simulink model "naibaoDSTBC_42"  (R2018a)
settings: Solver=VariableStepAuto  StartTime=0.0  StopTime=1  RelTol=1e-3
model workspace (MAT data in the model file):
  FrameLength = 100
  SampleTime = 0.001
  maxNumBits = 100000000
  maxNumErrs = 1000
undefined symbols (not defined in the file): doppler
libraries: commchan3 x9, commrandsrc3 x1, commsink2 x1
settings Model: Creator=myste  LastModifiedBy=myste

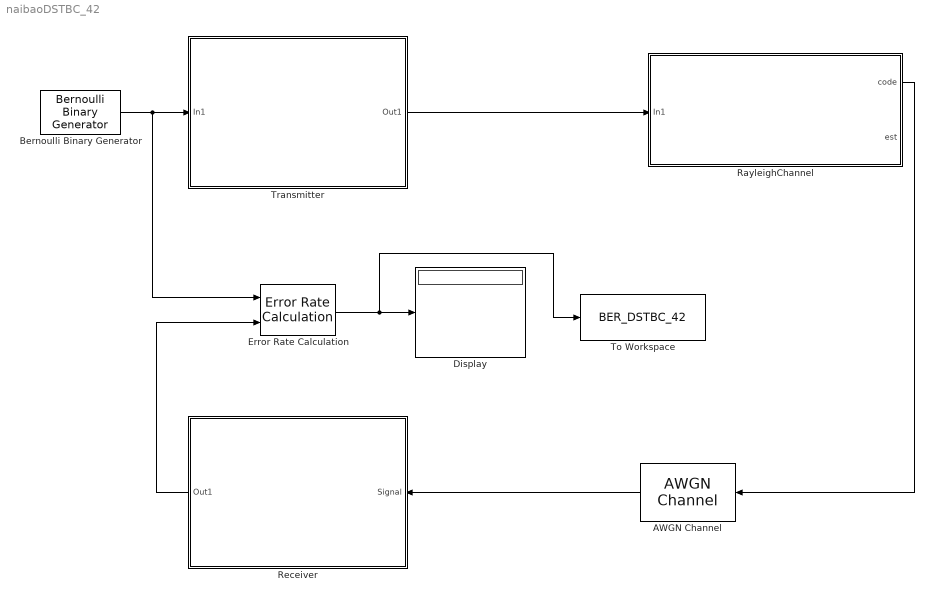
== system naibaoDSTBC_42 ==
  AWGN Channel : commchan3/AWGN Channel  InputProcessing=Columns as channels (frame based)  seed=3472  noiseMode="Signal to noise ratio  (Eb/No)"  EbNodB=EbNo  EsNodB=10  SNRdB=10  bitsPerSym=1  Ps=1  Tsym=SampleTime*1/2  variance=1
  Bernoulli Binary Generator : commrandsrc3/Bernoulli Binary Generator  ProbabilityOfZero=0.5  SeedSource=Auto  Seed=1983  SampleTime=SampleTime  SamplesPerFrame=FrameLength  OutputDataType=boolean  SimulateUsing=Interpreted execution
  Display : Display
  Error Rate Calculation : commsink2/Error Rate Calculation  N=0  st_delay=0  cp_mode=Entire frame  subframe=[]  PMode=Port  WsName=ErrorVec  RsMode2=off  stop=on  numErr=maxNumErrs  maxBits=maxNumBits
  RayleighChannel : Subsystem
  Receiver : Subsystem
  To Workspace : ToWorkspace  VariableName=BER_DSTBC_42  SampleTime=-1
      settings: MaxDataPoints=1  Save2DSignal=2-D array (concatenate along first dimension)
  Transmitter : Subsystem
  wires:
  Bernoulli Binary Generator/1 -> Error Rate Calculation/1, Transmitter/1(In1)
  Transmitter/1(Out1) -> RayleighChannel/1(In1)
  Receiver/1(Out1) -> Error Rate Calculation/2
  Error Rate Calculation/1 -> To Workspace/1, Display/1
  RayleighChannel/1(code) -> AWGN Channel/1
  AWGN Channel/1 -> Receiver/1(Signal)

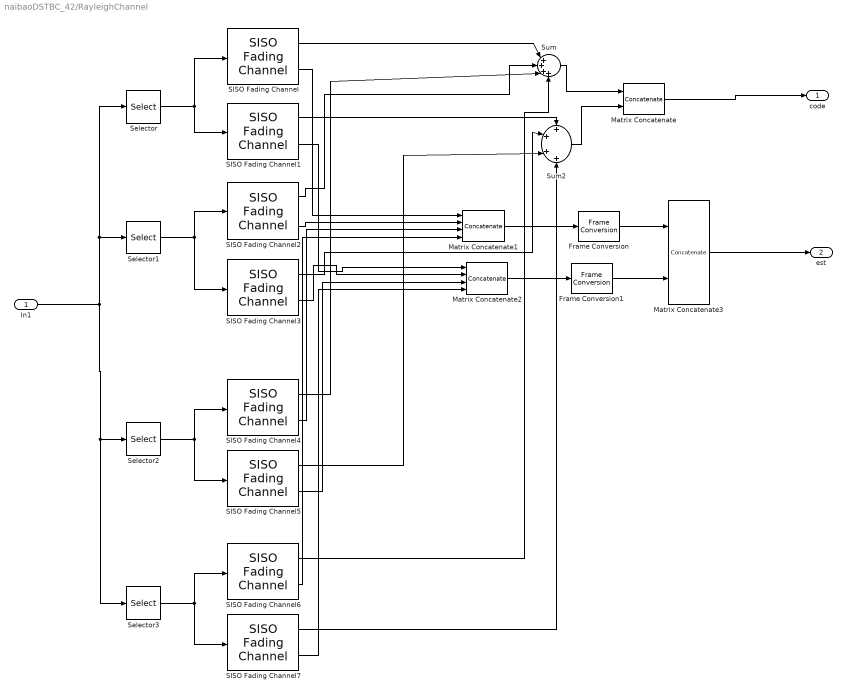
== system naibaoDSTBC_42/RayleighChannel ==
  In1 : Inport
  Frame Conversion : FrameConversion  OutFrame=Sample-based
  Frame Conversion1 : FrameConversion  OutFrame=Sample-based
  Matrix Concatenate : Concatenate  Mode=Multidimensional array  ConcatenateDimension=2
  Matrix Concatenate1 : Concatenate  NumInputs=4  Mode=Multidimensional array  ConcatenateDimension=2
  Matrix Concatenate2 : Concatenate  NumInputs=4  Mode=Multidimensional array  ConcatenateDimension=2
  Matrix Concatenate3 : Concatenate  Mode=Multidimensional array  ConcatenateDimension=3
  SISO Fading Channel : commchan3/SISO Fading Channel  InheritSampleRate=on  SampleRate=1  PathDelays=0  AveragePathGains=0  NormalizePathGains=on  FadingDistribution=Rayleigh  KFactor=3  DirectPathDopplerShift=0  DirectPathInitialPhase=0  MaximumDopplerShift=3  DopplerSpectrum=doppler('Jakes')  ChannelInterpolationMethod=Polyphase  RandomStream=mt19937ar with seed  RandomNumGenerator=mt19937ar  Seed=123  PathGainsOutputPort=on  ChannelFilterDelayOutputPort=off  SimulateUsing=Interpreted execution  Visualization=Off  PathsForDopplerDisplay=1  SamplesToDisplay=25%
      settings: SourceProductName=Communications System Toolbox
  SISO Fading Channel1 : commchan3/SISO Fading Channel  InheritSampleRate=on  SampleRate=1  PathDelays=0  AveragePathGains=0  NormalizePathGains=on  FadingDistribution=Rayleigh  KFactor=3  DirectPathDopplerShift=0  DirectPathInitialPhase=0  MaximumDopplerShift=3  DopplerSpectrum=doppler('Jakes')  ChannelInterpolationMethod=Polyphase  RandomStream=mt19937ar with seed  RandomNumGenerator=mt19937ar  Seed=73  PathGainsOutputPort=on  ChannelFilterDelayOutputPort=off  SimulateUsing=Interpreted execution  Visualization=Off  PathsForDopplerDisplay=1  SamplesToDisplay=25%
      settings: SourceProductName=Communications System Toolbox
  SISO Fading Channel2 : commchan3/SISO Fading Channel  InheritSampleRate=on  SampleRate=1  PathDelays=0  AveragePathGains=0  NormalizePathGains=on  FadingDistribution=Rayleigh  KFactor=3  DirectPathDopplerShift=0  DirectPathInitialPhase=0  MaximumDopplerShift=3  DopplerSpectrum=doppler('Jakes')  ChannelInterpolationMethod=Polyphase  RandomStream=mt19937ar with seed  RandomNumGenerator=mt19937ar  Seed=88  PathGainsOutputPort=on  ChannelFilterDelayOutputPort=off  SimulateUsing=Interpreted execution  Visualization=Off  PathsForDopplerDisplay=1  SamplesToDisplay=25%
      settings: SourceProductName=Communications System Toolbox
  SISO Fading Channel3 : commchan3/SISO Fading Channel  InheritSampleRate=on  SampleRate=1  PathDelays=0  AveragePathGains=0  NormalizePathGains=on  FadingDistribution=Rayleigh  KFactor=3  DirectPathDopplerShift=0  DirectPathInitialPhase=0  MaximumDopplerShift=3  DopplerSpectrum=doppler('Jakes')  ChannelInterpolationMethod=Polyphase  RandomStream=mt19937ar with seed  RandomNumGenerator=mt19937ar  Seed=95  PathGainsOutputPort=on  ChannelFilterDelayOutputPort=off  SimulateUsing=Interpreted execution  Visualization=Off  PathsForDopplerDisplay=1  SamplesToDisplay=25%
      settings: SourceProductName=Communications System Toolbox
  SISO Fading Channel4 : commchan3/SISO Fading Channel  InheritSampleRate=on  SampleRate=1  PathDelays=0  AveragePathGains=0  NormalizePathGains=on  FadingDistribution=Rayleigh  KFactor=3  DirectPathDopplerShift=0  DirectPathInitialPhase=0  MaximumDopplerShift=3  DopplerSpectrum=doppler('Jakes')  ChannelInterpolationMethod=Polyphase  RandomStream=mt19937ar with seed  RandomNumGenerator=mt19937ar  Seed=102  PathGainsOutputPort=on  ChannelFilterDelayOutputPort=off  SimulateUsing=Interpreted execution  Visualization=Off  PathsForDopplerDisplay=1  SamplesToDisplay=25%
      settings: SourceProductName=Communications System Toolbox
  SISO Fading Channel5 : commchan3/SISO Fading Channel  InheritSampleRate=on  SampleRate=1  PathDelays=0  AveragePathGains=0  NormalizePathGains=on  FadingDistribution=Rayleigh  KFactor=3  DirectPathDopplerShift=0  DirectPathInitialPhase=0  MaximumDopplerShift=3  DopplerSpectrum=doppler('Jakes')  ChannelInterpolationMethod=Polyphase  RandomStream=mt19937ar with seed  RandomNumGenerator=mt19937ar  Seed=143  PathGainsOutputPort=on  ChannelFilterDelayOutputPort=off  SimulateUsing=Interpreted execution  Visualization=Off  PathsForDopplerDisplay=1  SamplesToDisplay=25%
      settings: SourceProductName=Communications System Toolbox
  SISO Fading Channel6 : commchan3/SISO Fading Channel  InheritSampleRate=on  SampleRate=1  PathDelays=0  AveragePathGains=0  NormalizePathGains=on  FadingDistribution=Rayleigh  KFactor=3  DirectPathDopplerShift=0  DirectPathInitialPhase=0  MaximumDopplerShift=3  DopplerSpectrum=doppler('Jakes')  ChannelInterpolationMethod=Polyphase  RandomStream=mt19937ar with seed  RandomNumGenerator=mt19937ar  Seed=127  PathGainsOutputPort=on  ChannelFilterDelayOutputPort=off  SimulateUsing=Interpreted execution  Visualization=Off  PathsForDopplerDisplay=1  SamplesToDisplay=25%
      settings: SourceProductName=Communications System Toolbox
  SISO Fading Channel7 : commchan3/SISO Fading Channel  InheritSampleRate=on  SampleRate=1  PathDelays=0  AveragePathGains=0  NormalizePathGains=on  FadingDistribution=Rayleigh  KFactor=3  DirectPathDopplerShift=0  DirectPathInitialPhase=0  MaximumDopplerShift=3  DopplerSpectrum=doppler('Jakes')  ChannelInterpolationMethod=Polyphase  RandomStream=mt19937ar with seed  RandomNumGenerator=mt19937ar  Seed=164  PathGainsOutputPort=on  ChannelFilterDelayOutputPort=off  SimulateUsing=Interpreted execution  Visualization=Off  PathsForDopplerDisplay=1  SamplesToDisplay=25%
      settings: SourceProductName=Communications System Toolbox
  Selector : Selector  NumberOfDimensions=2  InputPortWidth=3  IndexOptions=Select all,Index vector (dialog)  Indices=[1 3],1  OutputSizes=1,1
  Selector1 : Selector  NumberOfDimensions=2  InputPortWidth=3  IndexOptions=Select all,Index vector (dialog)  Indices=[1 3],2  OutputSizes=1,1
  Selector2 : Selector  NumberOfDimensions=2  InputPortWidth=3  IndexOptions=Select all,Index vector (dialog)  Indices=[1 3],3  OutputSizes=1,1
  Selector3 : Selector  NumberOfDimensions=2  InputPortWidth=3  IndexOptions=Select all,Index vector (dialog)  Indices=[1 3],4  OutputSizes=1,1
  Sum : Sum  Inputs=|++++
  Sum2 : Sum  Inputs=++++
  code : Outport
  est : Outport  Port=2
  wires:
  In1/1 -> Selector3/1, Selector2/1, Selector/1, Selector1/1
  Selector/1 -> SISO Fading Channel/1, SISO Fading Channel1/1
  Selector1/1 -> SISO Fading Channel3/1, SISO Fading Channel2/1
  SISO Fading Channel/1 -> Sum/1
  SISO Fading Channel2/1 -> Sum/2
  SISO Fading Channel1/1 -> Sum2/1
  Sum/1 -> Matrix Concatenate/1
  Sum2/1 -> Matrix Concatenate/2
  SISO Fading Channel/2 -> Matrix Concatenate1/1
  SISO Fading Channel3/1 -> Sum2/2
  SISO Fading Channel2/2 -> Matrix Concatenate1/2
  SISO Fading Channel1/2 -> Matrix Concatenate2/1
  SISO Fading Channel3/2 -> Matrix Concatenate2/2
  Matrix Concatenate/1 -> code/1
  Matrix Concatenate1/1 -> Frame Conversion/1
  Matrix Concatenate2/1 -> Frame Conversion1/1
  Frame Conversion1/1 -> Matrix Concatenate3/2
  Frame Conversion/1 -> Matrix Concatenate3/1
  Matrix Concatenate3/1 -> est/1
  Selector2/1 -> SISO Fading Channel5/1, SISO Fading Channel4/1
  Selector3/1 -> SISO Fading Channel6/1, SISO Fading Channel7/1
  SISO Fading Channel4/1 -> Sum/3
  SISO Fading Channel6/1 -> Sum/4
  SISO Fading Channel5/1 -> Sum2/3
  SISO Fading Channel7/1 -> Sum2/4
  SISO Fading Channel4/2 -> Matrix Concatenate1/3
  SISO Fading Channel6/2 -> Matrix Concatenate1/4
  SISO Fading Channel5/2 -> Matrix Concatenate2/3
  SISO Fading Channel7/2 -> Matrix Concatenate2/4

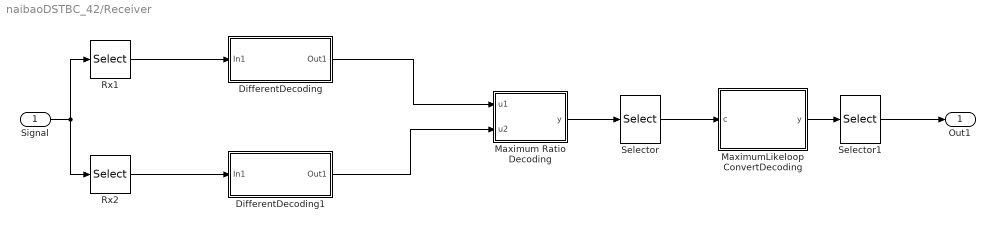
== system naibaoDSTBC_42/Receiver ==
  Signal : Inport
  DifferentDecoding : Subsystem
  DifferentDecoding1 : Subsystem
  Maximum Ratio Decoding : MATLAB Function  TreatAsAtomicUnit=on
  MaximumLikeloop ConvertDecoding : MATLAB Function  TreatAsAtomicUnit=on
  Rx1 : Selector  NumberOfDimensions=2  InputPortWidth=3  IndexOptions=Select all,Index vector (dialog)  Indices=[1 3],1  OutputSizes=1,1
  Rx2 : Selector  NumberOfDimensions=2  InputPortWidth=3  IndexOptions=Select all,Index vector (dialog)  Indices=[1 3],2  OutputSizes=1,1
  Selector : Selector  NumberOfDimensions=2  InputPortWidth=3  IndexOptions=Select all,Index vector (dialog)  Indices=[1 3],1  OutputSizes=1,1
  Selector1 : Selector  NumberOfDimensions=2  InputPortWidth=3  IndexOptions=Select all,Index vector (dialog)  Indices=[1 3],1  OutputSizes=1,1
  Out1 : Outport
  wires:
  Signal/1 -> Rx2/1, Rx1/1
  Rx1/1 -> DifferentDecoding/1(In1)
  Maximum Ratio Decoding/1(y) -> Selector/1
  Selector/1 -> MaximumLikeloop ConvertDecoding/1(c)
  DifferentDecoding/1(Out1) -> Maximum Ratio Decoding/1(u1)
  Rx2/1 -> DifferentDecoding1/1(In1)
  DifferentDecoding1/1(Out1) -> Maximum Ratio Decoding/2(u2)
  MaximumLikeloop ConvertDecoding/1(y) -> Selector1/1
  Selector1/1 -> Out1/1

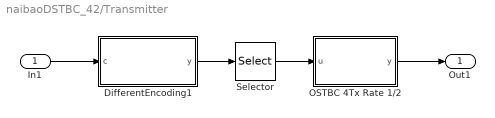
== system naibaoDSTBC_42/Transmitter ==
  In1 : Inport
  DifferentEncoding1 : MATLAB Function  TreatAsAtomicUnit=on
  OSTBC 4Tx Rate 1/2 : MATLAB Function  TreatAsAtomicUnit=on
  Selector : Selector  NumberOfDimensions=2  InputPortWidth=3  IndexOptions=Select all,Index vector (dialog)  Indices=[1 3],1  OutputSizes=1,1
  Out1 : Outport
  wires:
  In1/1 -> DifferentEncoding1/1(c)
  DifferentEncoding1/1(y) -> Selector/1
  Selector/1 -> OSTBC 4Tx Rate 1/2/1(u)
  OSTBC 4Tx Rate 1/2/1(y) -> Out1/1

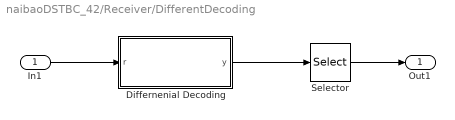
== system naibaoDSTBC_42/Receiver/DifferentDecoding ==
  In1 : Inport
  Differnenial Decoding : MATLAB Function  TreatAsAtomicUnit=on
  Selector : Selector  NumberOfDimensions=2  InputPortWidth=3  IndexOptions=Select all,Index vector (dialog)  Indices=[1 3],1  OutputSizes=1,1
  Out1 : Outport
  wires:
  Differnenial Decoding/1(y) -> Selector/1
  Selector/1 -> Out1/1
  In1/1 -> Differnenial Decoding/1(r)

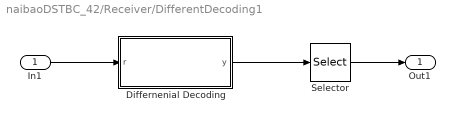
== system naibaoDSTBC_42/Receiver/DifferentDecoding1 ==
  In1 : Inport
  Differnenial Decoding : MATLAB Function  TreatAsAtomicUnit=on
  Selector : Selector  NumberOfDimensions=2  InputPortWidth=3  IndexOptions=Select all,Index vector (dialog)  Indices=[1 3],1  OutputSizes=1,1
  Out1 : Outport
  wires:
  Differnenial Decoding/1(y) -> Selector/1
  Selector/1 -> Out1/1
  In1/1 -> Differnenial Decoding/1(r)

== matlab function naibaoDSTBC_42/Transmitter/DifferentEncoding1 ==
  data: c input; y output
function y = DifferentEncoding4(c)
%将输入的码字按规则映射，之后差分编码
%% 设置参数
temp=complex(zeros(8,1));
%计数变量
num=0+0i;
%得到帧长
s = size(c);
%计算BPSK的长度
BPSK_Len = s(1);
%初始化系数序列
u = complex(zeros(BPSK_Len,1));
%初始编码
x1=1/2+0i;
x2=1/2+0i;
x3=1/2+0i;
x4=1/2+0i;
%初始化发送序列
y=complex(zeros(BPSK_Len+4,2));
y(1,1)=x1;
y(2,1)=x2;
y(3,1)=x3;
y(4,1)=x4;
%Naibao编码映射矩阵
w=[ 1 0 0 0           ; 0.5 -0.5 0.5 -0.5 ; 0.5 0.5 -0.5 -0.5 ; 0 0 0 -1           ;
    0.5 -0.5 -0.5 0.5 ; 0 -1 0 0          ; 0 0 -1 0          ; -0.5 -0.5 -0.5 -0.5;
    0.5 0.5 0.5 0.5   ; 0 0 1 0           ; 0 1 0 0           ; -0.5 0.5 0.5 -0.5  ;
    0 0 0 1           ; -0.5 -0.5 0.5 0.5 ; -0.5 0.5 -0.5 0.5 ; -1 0 0 0           ];
%小姐姐编码映射矩阵
w1=[ 1 0 0 0           ; 0.5 0.5 -0.5 0.5  ; 0.5 0.5 -0.5 0.5  ; 0 0.5 0 1          ;
    0.5 0.5 0.5 -0.5  ; 0    1   0    0   ; 0    0   1    0   ;-1/2 1/2 1/2 1/2    ;
    1/2 -1/2 -1/2 -1/2;0 0 -1/2 0         ; 0 -1 0 0          ;-1/2 -1/2 -1/2 1/2  ;
    0 0 0 -1          ;-1/2 1/2 -1/2 -1/2 ;-1/2 -1/2 0 -1/2   ;-1 0 0 0            ];
%% 差分编码    
for i=1:BPSK_Len/4
    V1=[x1,x2,x3,x4];
    V2=[-x2,x1,-x4,x3];
    V3=[-x3,x4,x1,-x2];
    V4=[-x4,-x3,x2,x1];
    Vc=[V1,conj(V1);V2,conj(V2);V3,conj(V3);V4,conj(V4)];
    %% 得到映射序列
%   num=double(c(4*i-3))+2^double(c(4*i-2))+4^double(c(4*i-1))+8^double(c(4*i));
    num=double(c(4*i))+2*double(c(4*i-1))+4*double(c(4*i-2))+8*double(c(4*i-3));
    for j=1:4
        u(4*(i-1)+j)=w(num+1,j);
    end
    %差分编码
    temp=u(4*(i-1)+1)*Vc(1,:) + u(4*(i-1)+2)*Vc(2,:) + u(4*(i-1)+3)*Vc(3,:) + u(4*(i-1)+4)*Vc(4,:);
    for j=1:4
        y(4*i+j,1)=temp(j);
    end
    %计算当前的基底
    x1=y(4*i+1,1);
    x2=y(4*i+2,1);
    x3=y(4*i+3,1);
    x4=y(4*i+4,1);
end

== matlab function naibaoDSTBC_42/Receiver/DifferentDecoding/Differnenial Decoding ==
  data: r input; y output
function y = DiffernenialDecoding(r)
%输出解码序列
%% 基本参数
% 获取帧长
s=size(r);
FrameLen=s(1);
% 初始化输出序列
y=complex(zeros( (FrameLen-8)/2,2));
%% 计算系数
for i=1:FrameLen/8-1
    % 接收到的当前分组符号
    R1=[r(8*(i-1)+1),r(8*(i-1)+2),r(8*(i-1)+3),r(8*(i-1)+4),r(8*(i-1)+5)',r(8*(i-1)+6)',r(8*(i-1)+7)',r(8*(i-1)+8)'];
    R2=[r(8*(i-1)+2),-r(8*(i-1)+1),-r(8*(i-1)+4),r(8*(i-1)+3),r(8*(i-1)+6)',-r(8*(i-1)+5)',-r(8*(i-1)+8)',r(8*(i-1)+7)'];
    R3=[r(8*(i-1)+3),r(8*(i-1)+4),-r(8*(i-1)+1),-r(8*(i-1)+2),r(8*(i-1)+7)',r(8*(i-1)+8)',-r(8*(i-1)+5)',-r(8*(i-1)+6)'];
    R4=[r(8*(i-1)+4),-r(8*(i-1)+3),r(8*(i-1)+2),-r(8*(i-1)+1),r(8*(i-1)+8)',-r(8*(i-1)+7)',r(8*(i-1)+6)',-r(8*(i-1)+5)'];
    % 接收到下一个分组符号
    Rxv=[r(8*i+1),r(8*i+2),r(8*i+3),r(8*i+4),r(8*i+5)',r(8*i+6)',r(8*i+7)',r(8*i+8)'];
    % 差分解码
    y(4*(i-1)+1,1)=(Rxv*R1');
    y(4*(i-1)+2,1)=(Rxv*R2');
    y(4*(i-1)+3,1)=(Rxv*R3');
    y(4*(i-1)+4,1)=(Rxv*R4');
end
y

== matlab function naibaoDSTBC_42/Receiver/DifferentDecoding1/Differnenial Decoding ==
  data: r input; y output
function y = DiffernenialDecoding(r)
%输出解码序列
%% 基本参数
% 获取帧长
s=size(r);
FrameLen=s(1);
% 初始化输出序列
y=complex(zeros( (FrameLen-8)/2,2));
%% 计算系数
for i=1:FrameLen/8-1
    % 接收到的当前分组符号
    R1=[r(8*(i-1)+1),r(8*(i-1)+2),r(8*(i-1)+3),r(8*(i-1)+4),r(8*(i-1)+5)',r(8*(i-1)+6)',r(8*(i-1)+7)',r(8*(i-1)+8)'];
    R2=[r(8*(i-1)+2),-r(8*(i-1)+1),-r(8*(i-1)+4),r(8*(i-1)+3),r(8*(i-1)+6)',-r(8*(i-1)+5)',-r(8*(i-1)+8)',r(8*(i-1)+7)'];
    R3=[r(8*(i-1)+3),r(8*(i-1)+4),-r(8*(i-1)+1),-r(8*(i-1)+2),r(8*(i-1)+7)',r(8*(i-1)+8)',-r(8*(i-1)+5)',-r(8*(i-1)+6)'];
    R4=[r(8*(i-1)+4),-r(8*(i-1)+3),r(8*(i-1)+2),-r(8*(i-1)+1),r(8*(i-1)+8)',-r(8*(i-1)+7)',r(8*(i-1)+6)',-r(8*(i-1)+5)'];
    % 接收到下一个分组符号
    Rxv=[r(8*i+1),r(8*i+2),r(8*i+3),r(8*i+4),r(8*i+5)',r(8*i+6)',r(8*i+7)',r(8*i+8)'];
    % 差分解码
    y(4*(i-1)+1,1)=(Rxv*R1');
    y(4*(i-1)+2,1)=(Rxv*R2');
    y(4*(i-1)+3,1)=(Rxv*R3');
    y(4*(i-1)+4,1)=(Rxv*R4');
end

== matlab function naibaoDSTBC_42/Transmitter/OSTBC 4Tx Rate 1//2 ==
  data: u input; y output
function y = naibaoOSTBC4(u)
%% 基本参数
%获取帧长
s=size(u);
FrameLen=s(1);
%初始化发射序列
y=complex(zeros(2*FrameLen,4));
%开始编码
for i=1:FrameLen/4
    x1=u(4*(i-1)+1);
    x2=u(4*(i-1)+2);
    x3=u(4*(i-1)+3);
    x4=u(4*(i-1)+4);
    y(8*(i-1)+1 : 8*(i-1)+8 ,1:4)=[x1,x2,x3,x4;
                                  -x2,x1,-x4,x3;
                                  -x3,x4,x1,-x2;
                                  -x4,-x3,x2,x1;
                                  x1',x2',x3',x4';
                                  -x2',x1',-x4',x3';
                                  -x3',x4',x1',-x2';
                                  -x4',-x3',x2',x1'];
end

== matlab function naibaoDSTBC_42/Receiver/Maximum Ratio Decoding ==
  data: u1 input; y output; u2 input
function y = mrd(u1,u2)
%两条信道完全对称,直接等增益合并
s=size(u1);
y=complex( zeros(s(1),2));
for i=1:s(1)
    y(i,1)=(u1(i)+u2(i))/2;
end

== matlab function naibaoDSTBC_42/Receiver/MaximumLikeloop ConvertDecoding ==
  data: c input; y output
function y  = MLC(c)
% 最大似然译码+逆映射
% 获取帧长
s=size(c);
FrameLen=s(1);
%初始化y
y=logical(zeros(FrameLen,2)); %#ok<LOGL>
%% 最大似然译码+逆映射
% naibao编码矩阵
allowcode=[ 1 0 0 0           ; 0.5 -0.5 0.5 -0.5 ; 0.5 0.5 -0.5 -0.5 ; 0 0 0 -1           ;
    0.5 -0.5 -0.5 0.5 ; 0 -1 0 0          ; 0 0 -1 0          ; -0.5 -0.5 -0.5 -0.5;
    0.5 0.5 0.5 0.5   ; 0 0 1 0           ; 0 1 0 0           ; -0.5 0.5 0.5 -0.5  ;
    0 0 0 1           ; -0.5 -0.5 0.5 0.5 ; -0.5 0.5 -0.5 0.5 ; -1 0 0 0           ];
%小姐姐编码矩阵
allowcode1=[ 1 0 0 0           ; 0.5 0.5 -0.5 0.5  ; 0.5 0.5 -0.5 0.5  ; 0 0.5 0 1          ;
    0.5 0.5 0.5 -0.5  ; 0    1   0    0   ; 0    0   1    0   ;-1/2 1/2 1/2 1/2    ;
    1/2 -1/2 -1/2 -1/2;0 0 -1/2 0         ; 0 -1 0 0          ;-1/2 -1/2 -1/2 1/2  ;
    0 0 0 -1          ;-1/2 1/2 -1/2 -1/2 ;-1/2 -1/2 0 -1/2   ;-1 0 0 0            ];
len=complex(zeros(16,1));
for i=1:FrameLen/4
    temp=[0+0i,1];
    for j=1:16
        len(j)=c(4*i-3)'*allowcode(j,1)+c(4*i-2)'*allowcode(j,2)+...
                    c(4*i-1)'*allowcode(j,3)+c(4*i)'*allowcode(j,4);
        if j==1 
            temp(1)=len(j);
        else
            if len(j)>temp(1)
                temp=[len(j),j];
            end
        end
    end
%     c(4*i-3)=allowcode(temp(2),1);
%     c(4*i-2)=allowcode(temp(2),2);
%     c(4*i-1)=allowcode(temp(2),3);
%     c(4*i-1)=allowcode(temp(2),4);
    num=dec2bin(real(temp(2)-1),4);
    y(4*i-3)=bin2dec(num(1));
    y(4*i-2)=bin2dec(num(2));
    y(4*i-1)=bin2dec(num(3));
    y(4*i)=bin2dec(num(4));
end
